simulink model "model_J"  (R2022a)
settings: Solver=VariableStepAuto  StartTime=0.0  StopTime=100  RelTol=1e-3
values from neighbouring files (symbols this model uses):
  A = [6, 7, -4, 8; 0, 9, 0, 15; 10, 13, -6, 19; 0, -6, 0, -9]    [task_2.m]
  B = [-8, 0; 4, 0; -6, 0; -2, 0]    [task_2.m]
  C = eye(4)    [task_2.m]
  D = zeros(4, 2)    [task_2.m]
  K_1 = -K_1    [task_2.m]
  K_2 = Y*inv(P)    [task_2.m]
  K_3 = Y*inv(P)    [task_2.m]
  Q_1 = 2*eye(4)    [task_2.m]
  R_1 = 2*eye(2)    [task_2.m]
  x0 = [1; -1; 1; -1]    [task_2.m]
undefined symbols (not defined in the file or in its folder): Q_2, Q_3, R_2, R_3
libraries: matrix_library x6
settings Model: Creator=vital  LastModifiedBy=Family
settings DebuggingCC: UnconnectedInputMsg=warning  UnconnectedOutputMsg=warning  UnconnectedLineMsg=warning
settings RTWCC: DLArmComputeVersion=19.05

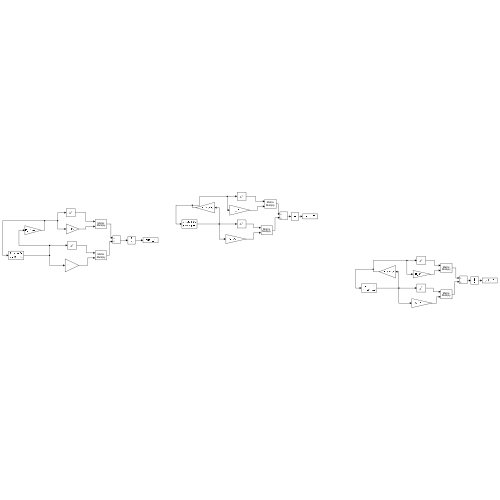
[thumbnail: Simulink's stored preview of the top-level diagram]
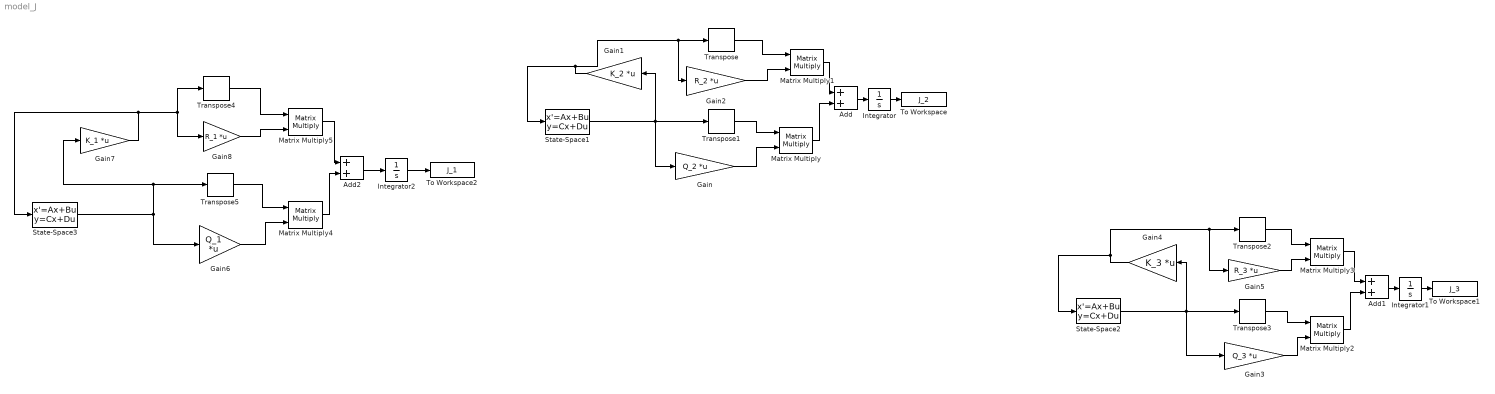
== system model_J ==
  Add : Sum
  Add1 : Sum
  Add2 : Sum
  Gain : Gain  Gain=Q_2  Multiplication=Matrix(K*u)
  Gain1 : Gain  Gain=K_2  Multiplication=Matrix(K*u) (u vector)
  Gain2 : Gain  Gain=R_2  Multiplication=Matrix(K*u)
  Gain3 : Gain  Gain=Q_3  Multiplication=Matrix(K*u)
  Gain4 : Gain  Gain=K_3  Multiplication=Matrix(K*u) (u vector)
  Gain5 : Gain  Gain=R_3  Multiplication=Matrix(K*u)
  Gain6 : Gain  Gain=Q_1  Multiplication=Matrix(K*u)
  Gain7 : Gain  Gain=K_1  Multiplication=Matrix(K*u) (u vector)
  Gain8 : Gain  Gain=R_1  Multiplication=Matrix(K*u)
  Integrator : Integrator
  Integrator1 : Integrator
  Integrator2 : Integrator
  Matrix Multiply{,1..5} (6 alike) : Product  Multiplication=Matrix(*)
  State-Space1 : StateSpace  A=A  B=B  C=C  D=D  InitialCondition=x0  ParameterTunability=Unconstrained
  State-Space2 : StateSpace  A=A  B=B  C=C  D=D  InitialCondition=x0  ParameterTunability=Unconstrained
  State-Space3 : StateSpace  A=A  B=B  C=C  D=D  InitialCondition=x0  ParameterTunability=Unconstrained
  To Workspace : ToWorkspace  VariableName=J_2  SaveFormat=Timeseries  SampleTime=0.0001
  To Workspace1 : ToWorkspace  VariableName=J_3  SaveFormat=Timeseries  SampleTime=0.0001
  To Workspace2 : ToWorkspace  VariableName=J_1  SaveFormat=Timeseries  SampleTime=0.0001
  Transpose{,1..5} (6 alike) : matrix_library/Transpose
      settings: SourceProductBaseCode=SL
  wires:
  State-Space1/1 -> Gain1/1, Gain/1, Transpose1/1
  Gain2/1 -> Matrix Multiply1/2
  Transpose/1 -> Matrix Multiply1/1
  Transpose1/1 -> Matrix Multiply/1
  Gain/1 -> Matrix Multiply/2
  Matrix Multiply/1 -> Add/2
  Matrix Multiply1/1 -> Add/1
  Gain1/1 -> Gain2/1, Transpose/1, State-Space1/1
  Add/1 -> Integrator/1
  Integrator/1 -> To Workspace/1
  Gain5/1 -> Matrix Multiply3/2
  Transpose2/1 -> Matrix Multiply3/1
  Gain3/1 -> Matrix Multiply2/2
  Transpose3/1 -> Matrix Multiply2/1
  Matrix Multiply3/1 -> Add1/1
  Integrator1/1 -> To Workspace1/1
  Add1/1 -> Integrator1/1
  Matrix Multiply2/1 -> Add1/2
  State-Space2/1 -> Gain4/1, Gain3/1, Transpose3/1
  Gain4/1 -> Gain5/1, Transpose2/1, State-Space2/1
  Gain8/1 -> Matrix Multiply5/2
  Transpose4/1 -> Matrix Multiply5/1
  Gain6/1 -> Matrix Multiply4/2
  Transpose5/1 -> Matrix Multiply4/1
  Matrix Multiply5/1 -> Add2/1
  Integrator2/1 -> To Workspace2/1
  Add2/1 -> Integrator2/1
  Matrix Multiply4/1 -> Add2/2
  State-Space3/1 -> Gain7/1, Transpose5/1, Gain6/1
  Gain7/1 -> Transpose4/1, Gain8/1, State-Space3/1
